simulink model "model"  (R2019b)
settings: Solver=VariableStepAuto  StartTime=0.0  StopTime=10.0  RelTol=1e-3
values from neighbouring files (symbols this model uses):
  alfa = alfa_beg    (= 1)    [param.m]
  beta = beta_beg    (= 1)    [param.m]
  cc = 15000    [param.m]
  cw = 200000    [param.m]
  dc = 200    [param.m]
  dw = 10    [param.m]
  k = k_beg    (= 1)    [param.m]
  mc = 250    [param.m]
  mw = 30    [param.m]
  xc = 0.5    [param.m]
  xw = 0.2    [param.m]
settings Model: Creator=Łukasz  LastModifiedBy=Łukasz

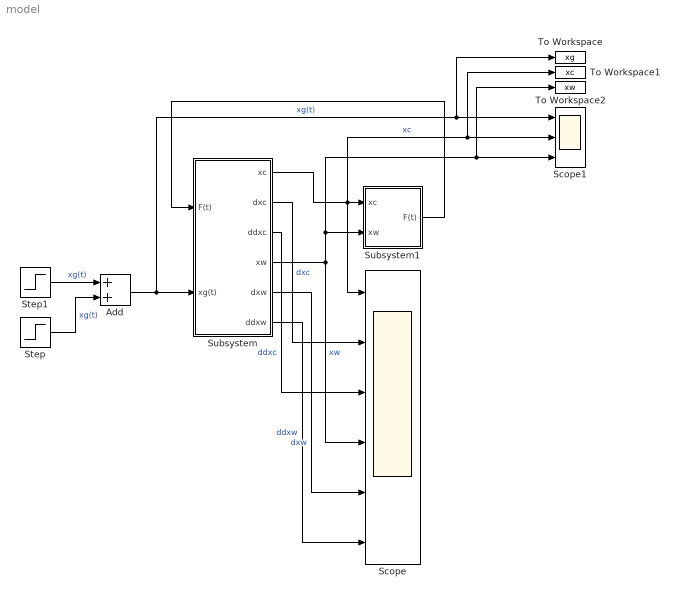
== system model ==
  Add : Sum
  Scope : Scope  NumInputPorts=6
  Scope1 : Scope  NumInputPorts=3
  Step : Step  Time=6  After=-0.5  SampleTime=0
  Step1 : Step  Time=2  After=0.5  SampleTime=0
  Subsystem : Subsystem
  Subsystem1 : Subsystem
  To Workspace : ToWorkspace  VariableName=xg  SaveFormat=Timeseries  SampleTime=-1
  To Workspace1 : ToWorkspace  VariableName=xc  SaveFormat=Timeseries  SampleTime=-1
  To Workspace2 : ToWorkspace  VariableName=xw  SaveFormat=Timeseries  SampleTime=-1
  wires:
  Subsystem/1(xc) -> Scope1/2, To Workspace1/1, Scope/1, Subsystem1/1(xc)  "xc"
  Subsystem/4(xw) -> Scope1/3, To Workspace2/1, Subsystem1/2(xw), Scope/4  "xw"
  Subsystem1/1(F(t)) -> Subsystem/1(F(t))
  Add/1 -> Scope1/1, To Workspace/1, Subsystem/2(xg(t))  "xg(t)"
  Subsystem/2(dxc) -> Scope/2  "dxc"
  Subsystem/3(ddxc) -> Scope/3  "ddxc"
  Subsystem/5(dxw) -> Scope/5  "dxw"
  Subsystem/6(ddxw) -> Scope/6  "ddxw"
  Step1/1 -> Add/1  "xg(t)"
  Step/1 -> Add/2  "xg(t)"

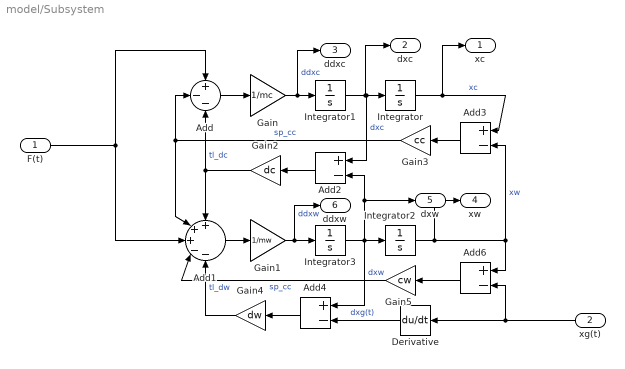
== system model/Subsystem ==
  F(t) : Inport
  xg(t) : Inport  Port=2
  Add : Sum  Inputs=+--
  Add1 : Sum  Inputs=+++--
  Add{2..4,6} (4 alike) : Sum  Inputs=+-
  Derivative : Derivative
  Gain : Gain  Gain=1/mc
  Gain1 : Gain  Gain=1/mw
  Gain2 : Gain  Gain=dc
  Gain3 : Gain  Gain=cc
  Gain4 : Gain  Gain=dw
  Gain5 : Gain  Gain=cw
  Integrator : Integrator  InitialCondition=xc
  Integrator1 : Integrator
  Integrator2 : Integrator  InitialCondition=xw
  Integrator3 : Integrator
  xc : Outport
  dxc : Outport  Port=2
  ddxc : Outport  Port=3
  xw : Outport  Port=4
  dxw : Outport  Port=5
  ddxw : Outport  Port=6
  wires:
  Integrator3/1 -> Add4/1, dxw/1, Add2/2, Integrator2/1  "dxw"
  Add6/1 -> Gain5/1
  Add1/1 -> Gain1/1
  Gain/1 -> ddxc/1, Integrator1/1  "ddxc"
  Gain1/1 -> ddxw/1, Integrator3/1  "ddxw"
  Integrator1/1 -> dxc/1, Add2/1, Integrator/1  "dxc"
  F(t)/1 -> Add1/3, Add/1
  Integrator2/1 -> xw/1, Add6/1, Add3/2  "xw"
  Add/1 -> Gain/1
  Add2/1 -> Gain2/1
  Gain3/1 -> Add/2, Add1/2  "sp_cc"
  Gain2/1 -> Add1/1, Add/3  "tl_dc"
  Gain5/1 -> Add1/4  "sp_cc"
  Gain4/1 -> Add1/5  "tl_dw"
  xg(t)/1 -> Add6/2, Derivative/1
  Derivative/1 -> Add4/2  "dxg(t)"
  Add4/1 -> Gain4/1
  Integrator/1 -> xc/1, Add3/1  "xc"
  Add3/1 -> Gain3/1

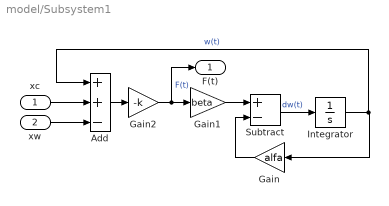
== system model/Subsystem1 ==
  xc : Inport
  xw : Inport  Port=2
  Add : Sum  Inputs=++-
  Gain : Gain  Gain=alfa
  Gain1 : Gain  Gain=beta
  Gain2 : Gain  Gain=-k
  Integrator : Integrator
  Subtract : Sum  Inputs=+-
  F(t) : Outport
  wires:
  Subtract/1 -> Integrator/1  "dw(t)"
  Integrator/1 -> Add/1, Gain/1  "w(t)"
  xc/1 -> Add/2
  Add/1 -> Gain2/1
  Gain1/1 -> Subtract/1
  Gain/1 -> Subtract/2
  Gain2/1 -> F(t)/1, Gain1/1  "F(t)"
  xw/1 -> Add/3
